simulink model "Harness_Angle"  (R2018a)
settings: Solver=VariableStepAuto  StartTime=0.0  StopTime=10.0  RelTol=1e-3
undefined symbols (not defined in the file): Automatic_Test
libraries: mciapi_libbrowser x1
settings Model: Creator=PATILMP  LastModifiedBy=PATILMP

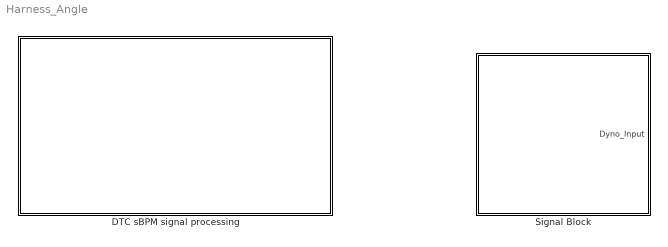
== system Harness_Angle ==
  DTC sBPM signal processing : Subsystem
  Signal Block : Subsystem

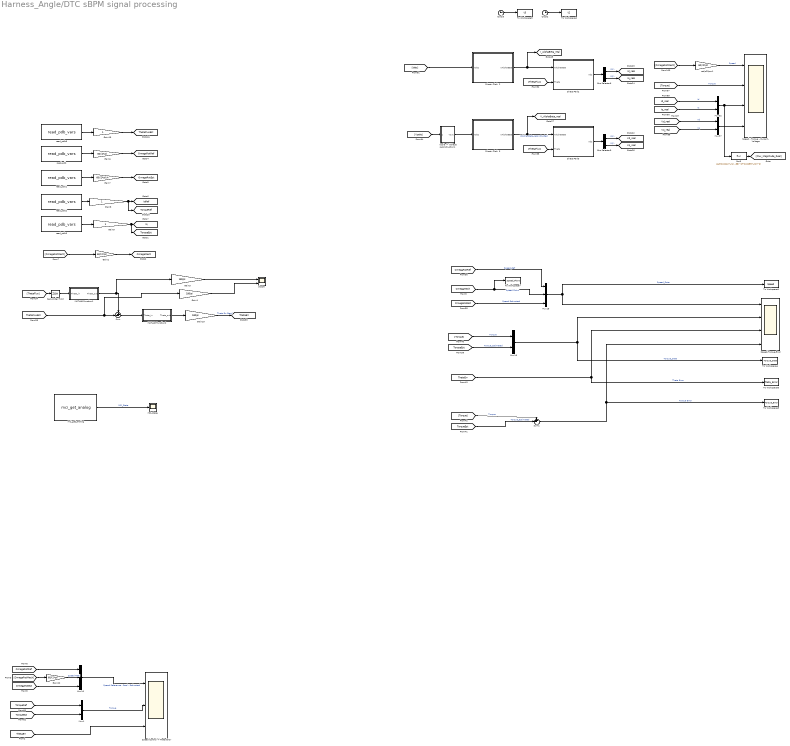
== system Harness_Angle/DTC sBPM signal processing ==
  Bus Selector6 : BusSelector  OutputSignals=D,Q
  Bus Selector9 : BusSelector  OutputSignals=D,Q
  Clock2 : Clock
  Clock3 : Clock
  Direct  Clark  2 : MATLAB Function  TreatAsAtomicUnit=on  SystemSampleTime=SystemSampleTime  mask{SystemSampleTime=-1}
      mask prompts: SystemSampleTime "Simulink:blkprm_prompts:AllBlksSampleTime"
  Direct  Clark  3 : MATLAB Function  TreatAsAtomicUnit=on  SystemSampleTime=SystemSampleTime  mask{SystemSampleTime=-1}
      mask prompts: SystemSampleTime "Simulink:blkprm_prompts:AllBlksSampleTime"
  Direct Park2 : MATLAB Function  TreatAsAtomicUnit=on  SystemSampleTime=SystemSampleTime  mask{SystemSampleTime=-1}
      mask prompts: SystemSampleTime "Simulink:blkprm_prompts:AllBlksSampleTime"
  Direct Park3 : MATLAB Function  TreatAsAtomicUnit=on  SystemSampleTime=SystemSampleTime  mask{SystemSampleTime=-1}
      mask prompts: SystemSampleTime "Simulink:blkprm_prompts:AllBlksSampleTime"
  Fcn5 : Fcn  Expr=sqrt((0.0212*u(1)+0.0688)^2+(0.0299*u(2))^2)
  Gain1 : Gain  Gain=180/pi
  Gain15 : Gain  OutDataTypeStr=double  RndMeth=Zero
  Gain19 : Gain  Gain=180/pi
  Gain2 : Gain  Gain=60/(2*pi)  RndMeth=Round
  Gain22 : Gain  Gain=60/(2*pi)  RndMeth=Round
  Gain3 : Gain  Gain=180/pi
  Gain6 : Gain  Gain=60/(2*pi)  OutDataTypeStr=double  RndMeth=Zero
  Gain7 : Gain  Gain=60/(2*pi)/4  OutDataTypeStr=double  RndMeth=Zero
  Gain8 : Gain  OutDataTypeStr=double  RndMeth=Zero
  Gain9 : Gain  OutDataTypeStr=double  RndMeth=Zero
  MATLAB Function1 : MATLAB Function  TreatAsAtomicUnit=on
  MATLAB Function2 : MATLAB Function  TreatAsAtomicUnit=on
  MCI_State : Scope
  Mux{1,16,32,37} (4 alike) : Mux  Inputs=2
  Mux10 : Mux  Inputs=3
  Mux15 : Mux  Inputs=3
  Scope : Scope  NumInputPorts=2
  Speed - Torque - Current - Voltage : Scope  NumInputPorts=4
  Speed Control + Theta Error : Scope  NumInputPorts=3
  Speed-Torque-Error : Scope  NumInputPorts=4
  Sum : Sum  Inputs=+-|
  Sum1 : Sum  Inputs=+-|
  To Workspace1 : ToWorkspace  VariableName=Speed  SaveFormat=Timeseries  SampleTime=-1
  To Workspace2 : ToWorkspace  VariableName=t2  SampleTime=-1
      settings: Save2DSignal=2-D array (concatenate along first dimension)
  To Workspace3 : ToWorkspace  VariableName=t3  SampleTime=-1
      settings: Save2DSignal=2-D array (concatenate along first dimension)
  To Workspace4 : ToWorkspace  VariableName=Torque_Data  SaveFormat=Timeseries  SampleTime=-1
  To Workspace5 : ToWorkspace  VariableName=Torque_Error  SaveFormat=Timeseries  SampleTime=-1
  To Workspace6 : ToWorkspace  VariableName=Theta_Error  SaveFormat=Timeseries  SampleTime=-1
  To Workspace7 : ToWorkspace  VariableName=Speed_Plant  SaveFormat=Timeseries  SampleTime=-1
  "Vpole -> Vphase reconstruction1" : MATLAB Function  TreatAsAtomicUnit=on
  Zero-Order Hold : ZeroOrderHold  SampleTime=0.000125
  mci_get_analog : S-Function  FunctionName=mci_get_analog  Parameters=read_data, choose_read_data  SFunctionDeploymentMode=off  EnableBusSupport=off  mask{choose_read_data=MCI_AI_INTERNAL_MCI_STATE, read_data=24}
      mask prompts: choose_read_data "Data to read"
      mask TypeOptions choose_read_data: MCI_AI_TARGET_SPEED_RPM_S16 | MCI_AI_SPEED_REFERENCE_RPM_S16 | MCI_AI_ACTUAL_SPEED_S16 | MCI_AI_SPEED_ERROR_RPM_S16 | MCI_AI_MEAN_SPEED_S16 | MCI_AI_RMS_MOTOR_CURRENT_S16 | MCI_AI_ACTIVE_POWER_S16 | MCI_AI_SHAFT_POWER_S16 | MCI_AI_MOTOR_TEMP_S16 | MCI_AI_STATOR_TEMP_S16 | MCI_AI_LOAD_TORQUE_S16 | MCI_AI_SHAFT_POSITION_DEG_S16 | MCI_AI_BUS_CURRENT_S16 | MCI_AI_BUS_VOLTAGE_S16 | MCI_AI_INVERTER_TEMP_S16 | MCI_AI_INVERTER_TEMP_RAW_DATA | MCI_AI_VOLTAGE_PHASE_A_S16 | MCI_AI_VOLTAGE_PHASE_B_S16 | MCI_AI_VOLTAGE_PHASE_C_S16 | MCI_AI_SPEED_LOOP_GAIN_TABLE_INDEX | MCI_AI_CURR_PHASE_A_S16 | MCI_AI_CURR_PHASE_B_S16 | MCI_AI_CURR_PHASE_C_S16 | MCI_AI_STATOR_RESISTANCE_S16 | MCI_AI_INTERNAL_MCI_STATE
      mask Callback read_data:
      | rd = get_param(gcb,'choose_read_data');
      | poenum = strcat('MCI_AI_TYPE.',rd);
      | i_32 = eval(['int32(' poenum ')']);
      | set_param(gcb,'read_data',int2str(i_32));
      mask Display:
      | disp = regexp(choose_read_data, 'MCI_AI_', 'split');
      | port_label('output', 1, disp{2});
  rad/s2Rpm1 : Gain  Gain=60/(2*pi)
  read_pdb : S-Function  FunctionName=read_pdb_vars  Parameters=vstring  SFunctionDeploymentMode=off  EnableBusSupport=off  mask{vstring=Mcl_IO.Speed_Rot_Ref}
      mask prompts: vstring "Variable to read"
      mask Display:
      | disp = vstring;
      | port_label('output', 1, disp);
  read_pdb1 : S-Function  FunctionName=read_pdb_vars  Parameters=vstring  SFunctionDeploymentMode=off  EnableBusSupport=off  mask{vstring=Mcl_Quantities.Speed_Rot}
      mask prompts: vstring "Variable to read"
      mask Display:
      | disp = vstring;
      | port_label('output', 1, disp);
  read_pdb2 : S-Function  FunctionName=read_pdb_vars  Parameters=vstring  SFunctionDeploymentMode=off  EnableBusSupport=off  mask{vstring=Mcl_Quantities.Torque_Ref}
      mask prompts: vstring "Variable to read"
      mask Display:
      | disp = vstring;
      | port_label('output', 1, disp);
  read_pdb3 : S-Function  FunctionName=read_pdb_vars  Parameters=vstring  SFunctionDeploymentMode=off  EnableBusSupport=off  mask{vstring=Mcl_Quantities.Torque}
      mask prompts: vstring "Variable to read"
      mask Display:
      | disp = vstring;
      | port_label('output', 1, disp);
  read_pdb8 : S-Function  FunctionName=read_pdb_vars  Parameters=vstring  SFunctionDeploymentMode=off  EnableBusSupport=off  mask{vstring=Mcl_Quantities.Rotor_Position}
      mask prompts: vstring "Variable to read"
      mask Display:
      | disp = vstring;
      | port_label('output', 1, disp);
  tag scope: I_AlphaBeta_real=global, Id_real=global, Iq=global, IqRef=global, Iq_real=global, OmegaMech=global, OmegaRotEst=global, OmegaRotRef=global, ThetaErr=global, ThetaFluxEst=global, TorqueEst=global, TorqueRef=global, V_AlphaBeta_real=global, Vd_real=global, Vq_real=global
  wires:
  [ThetaFlux] -> Zero-Order Hold/1
  MATLAB Function1/1(Theta_out) -> Gain3/1, Sum/1
  Sum/1 -> MATLAB Function2/1(Theta_in)
  Gain19/1 -> [ThetaErr]  "Theta Err [deg]"
  MATLAB Function2/1(Theta_out) -> Gain19/1
  Zero-Order Hold/1 -> MATLAB Function1/1(Theta_in)
  [ThetaFluxEst] -> Gain1/1, Sum/2
  Bus Selector6/1 -> [Id_real]  "<D>"
  [Vpole] -> "Vpole -> Vphase reconstruction1"/1(Vpole)
  [Vq_real] -> Mux37/2  "Vq"
  Bus Selector6/2 -> [Iq_real]  "<Q>"
  "Vpole -> Vphase reconstruction1"/1(Vout) -> Direct  Clark  3/1(Xabc)
  [ThetaFlux] -> Direct Park3/2(Theta)
  Mux32/1 -> Fcn5/1, Speed - Torque - Current - Voltage/3
  Direct Park2/1(Xdq) -> Bus Selector6/1
  Clock2/1 -> To Workspace2/1
  [Iq_real] -> Mux32/2  "Iq"
  rad/s2Rpm1/1 -> Speed - Torque - Current - Voltage/1  "Speed"
  Mux37/1 -> Speed - Torque - Current - Voltage/4
  Clock3/1 -> To Workspace3/1
  [Iabc] -> Direct  Clark  2/1(Xabc)
  Bus Selector9/1 -> [Vd_real]  "<D>"
  [ThetaFlux] -> Direct Park2/2(Theta)
  [Torque] -> Speed - Torque - Current - Voltage/2  "Torque"
  [Id_real] -> Mux32/1  "Id"
  [Vd_real] -> Mux37/1  "Vd"
  Bus Selector9/2 -> [Vq_real]  "<Q>"
  Direct  Clark  3/1(XAlphaBeta) -> Direct Park3/1(XAlphaBeta), [V_AlphaBeta_real]  "Valpha_Beta_reconstructed"
  Direct Park3/1(Xdq) -> Bus Selector9/1
  Direct  Clark  2/1(XAlphaBeta) -> [I_AlphaBeta_real], Direct Park2/1(XAlphaBeta)
  [OmegaRotMech] -> rad/s2Rpm1/1
  Gain8/1 -> [TorqueRef], [IqRef]
  Gain9/1 -> [TorqueEst], [Iq]
  read_pdb/1 -> Gain6/1
  read_pdb8/1 -> Gain15/1
  Gain15/1 -> [ThetaFluxEst]
  read_pdb3/1 -> Gain9/1
  read_pdb2/1 -> Gain8/1
  Gain6/1 -> [OmegaRotRef]
  read_pdb1/1 -> Gain7/1
  Gain7/1 -> [OmegaRotEst]
  [TorqueEst] -> Mux1/2
  [TorqueRef] -> Mux1/1
  Mux1/1 -> Speed Control + Theta Error/2  "Torque"
  mci_get_analog/1 -> MCI_State/1  "MCI_State"
  Fcn5/1 -> [Flux_Magnitude_Real]
  Mux15/1 -> Speed-Torque-Error/1, To Workspace1/1  "Speed_Data"
  [TorqueEst] -> Sum1/2  "Torque_estimated"
  [TorqueEst] -> Mux16/2  "Torque_estimated"
  [Torque] -> Mux16/1  "Torque"
  Sum1/1 -> Speed-Torque-Error/4, To Workspace5/1  "Torque Error"
  [OmegaRotEst] -> Mux15/3  "Speed Estimated"
  [OmegaMech] -> To Workspace7/1, Mux15/2  "Speed Plant"
  [Torque] -> Sum1/1  "Torque"
  Mux16/1 -> To Workspace4/1, Speed-Torque-Error/2  "Torque_Data"
  [ThetaErr] -> To Workspace6/1, Speed-Torque-Error/3  "Theta Error"
  [OmegaRotRef] -> Mux15/1  "Speed_Ref"
  [OmegaRotEst] -> Mux10/3
  Gain22/1 -> Mux10/2  "Speed Real"
  [OmegaRotRef] -> Mux10/1
  Mux10/1 -> Speed Control + Theta Error/1  "Speed Reference - Real - Estimated"
  [OmegaRotMech] -> Gain22/1
  [ThetaErr] -> Speed Control + Theta Error/3
  Gain2/1 -> [OmegaMech]
  [OmegaRotMech] -> Gain2/1
  Gain1/1 -> Scope/2
  Gain3/1 -> Scope/1

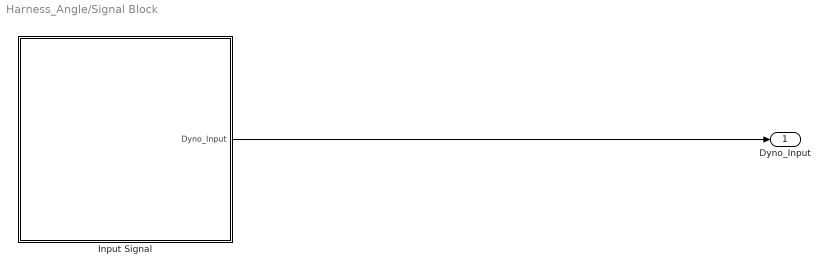
== system Harness_Angle/Signal Block ==
  Input Signal : Subsystem
  Dyno_Input : Outport
  wires:
  Input Signal/1(Dyno_Input) -> Dyno_Input/1

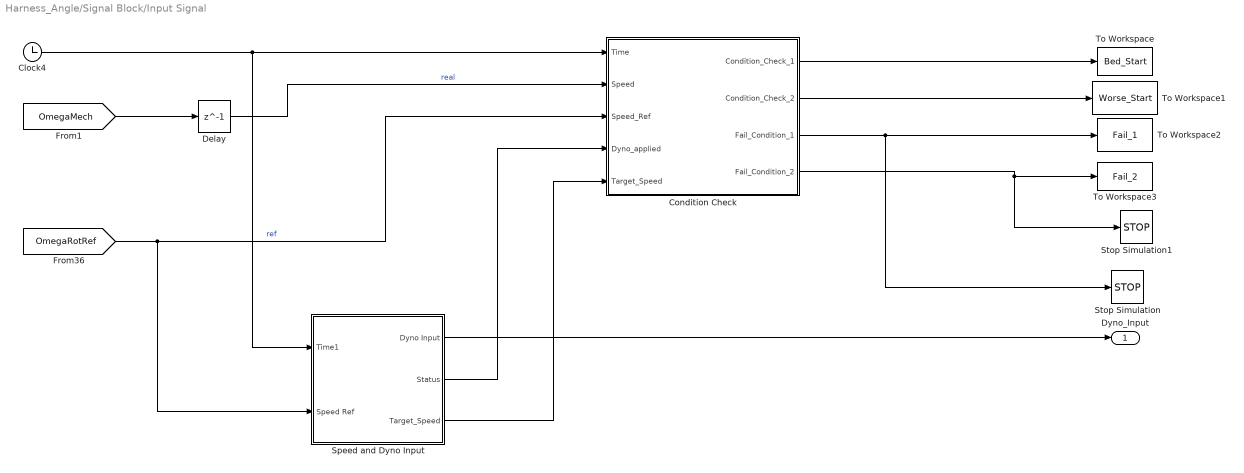
== system Harness_Angle/Signal Block/Input Signal ==
  Clock4 : Clock
  Condition Check : MATLAB Function  TreatAsAtomicUnit=on  mask(Condition Check){Speed_Tolerance=Automatic_Test.Speed_Tolerance, Para_time_check_1=Automatic_Test.Para_time_check_1, Para_time_check_2=Automatic_Test.Para_time_check_2, Para_time_check_3=Automatic_Test.Para_time_check_3, Speed_Tolerance_1=Automatic_Test.Speed_Tolerance_1}
      mask prompts: Speed_Tolerance "Speed Tolerance Value"; Speed_Tolerance_1 "Speed Tolerance Value_1"
      mask help: This block is used to check failure conditions.
  Delay : Delay  DelayLength=1
  Speed and Dyno Input : Subsystem
  Stop Simulation : Stop
  Stop Simulation1 : Stop
  To Workspace : ToWorkspace  VariableName=Bed_Start  SaveFormat=Timeseries  SampleTime=-1
  To Workspace1 : ToWorkspace  VariableName=Worse_Start  SaveFormat=Timeseries  SampleTime=-1
  To Workspace2 : ToWorkspace  VariableName=Fail_1  SaveFormat=Timeseries  SampleTime=-1
  To Workspace3 : ToWorkspace  VariableName=Fail_2  SaveFormat=Timeseries  SampleTime=-1
  Dyno_Input : Outport
  wires:
  [OmegaMech] -> Delay/1
  Delay/1 -> Condition Check/2(Speed)  "real"
  [OmegaRotRef] -> Speed and Dyno Input/2(Speed Ref), Condition Check/3(Speed_Ref)  "ref"
  Speed and Dyno Input/1(Dyno Input) -> Dyno_Input/1
  Condition Check/1(Condition_Check_1) -> To Workspace/1
  Condition Check/2(Condition_Check_2) -> To Workspace1/1
  Condition Check/3(Fail_Condition_1) -> Stop Simulation/1, To Workspace2/1
  Clock4/1 -> Condition Check/1(Time), Speed and Dyno Input/1(Time1)
  Condition Check/4(Fail_Condition_2) -> Stop Simulation1/1, To Workspace3/1
  Speed and Dyno Input/2(Status) -> Condition Check/4(Dyno_applied)
  Speed and Dyno Input/3(Target_Speed) -> Condition Check/5(Target_Speed)

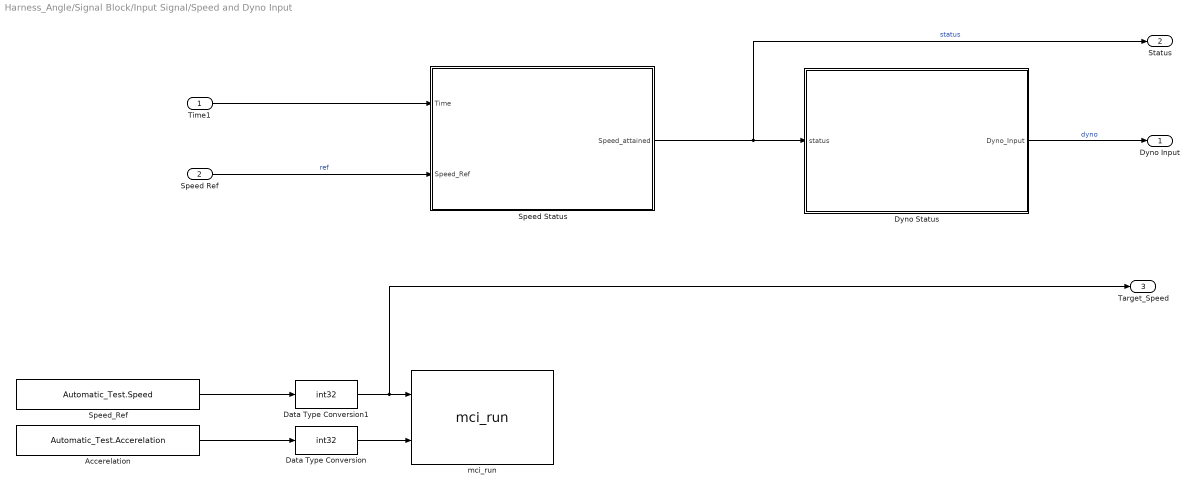
== system Harness_Angle/Signal Block/Input Signal/Speed and Dyno Input ==
  Time1 : Inport
  Speed Ref : Inport  Port=2
  Accerelation : Constant  Value=Automatic_Test.Accerelation
  Data Type Conversion : DataTypeConversion  OutDataTypeStr=int32
  Data Type Conversion1 : DataTypeConversion  OutDataTypeStr=int32
  Dyno Status : MATLAB Function  TreatAsAtomicUnit=on  mask(Speed Status){Dyno_Load=Automatic_Test.Dyno_Load}
      mask help: Once this block gets the active high signal from the speed ref status block, dyno load torque input gets activated and given as output.
  Speed Status : MATLAB Function  TreatAsAtomicUnit=on  mask(Speed Status){Status_Time_Check=Automatic_Test.Status_Time_Check}
      mask prompts: Status_Time_Check "Status Time Check"
      mask help: This Matlab function block is used to get the status of reference and estimated speed.
  Speed_Ref : Constant  Value=Automatic_Test.Speed
  mci_run : mciapi_libbrowser/mci_run  SFunctionModules=''
      settings: SourceProductName=Sim Arch
  Dyno Input : Outport
  Status : Outport  Port=2
  Target_Speed : Outport  Port=3
  wires:
  Accerelation/1 -> Data Type Conversion/1
  Data Type Conversion/1 -> mci_run/2
  Time1/1 -> Speed Status/1(Time)
  Speed Status/1(Speed_attained) -> Status/1, Dyno Status/1(status)  "status"
  Speed Ref/1 -> Speed Status/2(Speed_Ref)  "ref"
  Data Type Conversion1/1 -> Target_Speed/1, mci_run/1
  Dyno Status/1(Dyno_Input) -> Dyno Input/1  "dyno"
  Speed_Ref/1 -> Data Type Conversion1/1

== matlab function Harness_Angle/DTC sBPM signal processing/Direct  Clark  2 ==
  data: XAlphaBeta output Bus: XAlphaBetaBus; Xabc input Bus: XabcBus
function XAlphaBeta = DirectClark(Xabc)

XAlphaBeta.Alpha = Xabc.A;
XAlphaBeta.Beta =  sqrt(3)/3*(Xabc.A+2*Xabc.B);

== matlab function Harness_Angle/DTC sBPM signal processing/Direct  Clark  3 ==
  data: XAlphaBeta output Bus: XAlphaBetaBus; Xabc input Bus: XabcBus
function XAlphaBeta = DirectClark(Xabc)

XAlphaBeta.Alpha = Xabc.A;
XAlphaBeta.Beta =  sqrt(3)/3*(Xabc.A+2*Xabc.B);

== matlab function Harness_Angle/DTC sBPM signal processing/Direct Park2 ==
  data: XAlphaBeta input Bus: XAlphaBetaBus; Xdq output Bus: XdqBus; Theta input
function Xdq = DirectPark(XAlphaBeta,Theta)

Xdq.D  =  XAlphaBeta.Alpha*cos(Theta) + XAlphaBeta.Beta*sin(Theta);
Xdq.Q  = -XAlphaBeta.Alpha*sin(Theta) + XAlphaBeta.Beta*cos(Theta);

== matlab function Harness_Angle/DTC sBPM signal processing/Direct Park3 ==
  data: XAlphaBeta input Bus: XAlphaBetaBus; Xdq output Bus: XdqBus; Theta input
function Xdq = DirectPark(XAlphaBeta,Theta)

Xdq.D  =  XAlphaBeta.Alpha*cos(Theta) + XAlphaBeta.Beta*sin(Theta);
Xdq.Q  = -XAlphaBeta.Alpha*sin(Theta) + XAlphaBeta.Beta*cos(Theta);

== matlab function Harness_Angle/DTC sBPM signal processing/MATLAB Function1 ==
  data: Theta_in input; Theta_out output
function Theta_out = fcn(Theta_in)
%#codegen

if(Theta_in > pi)||(Theta_in < -pi)
    
    Resto_pi =  mod(Theta_in, pi);
    Resto_2pi =  mod(Theta_in, 2*pi);
    
    
    if(Resto_pi ~= Resto_2pi)
    Theta_out = -pi+Resto_pi;
    else
    Theta_out = Resto_pi;    
    end
 
else
    
    Theta_out = Theta_in;
    
end

== matlab function Harness_Angle/DTC sBPM signal processing/MATLAB Function2 ==
  data: Theta_in input; Theta_out output
function Theta_out = fcn(Theta_in)
%#codegen

if(Theta_in > pi)||(Theta_in < -pi)
    
    Resto_pi =  mod(Theta_in, pi);
    Resto_2pi =  mod(Theta_in, 2*pi);
    
    
    if(Resto_pi ~= Resto_2pi)
    Theta_out = -pi+Resto_pi;
    else
    Theta_out = Resto_pi;    
    end
 
else
    
    Theta_out = Theta_in;
    
end

== matlab function Harness_Angle/DTC sBPM signal processing/Vpole -> Vphase reconstruction1 ==
  data: Vpole input Bus: XabcBus size=1; Vout output Bus: XabcBus
function Vout   = Vrec2(Vpole)

Va = Vpole.A;
Vb = Vpole.B;
Vc = Vpole.C;

Vn = (Va + Vb + Vc)/3;

Vphase.A = Va - Vn;
Vphase.B = Vb - Vn;
Vphase.C = Vc - Vn;

Vline.A = Va - Vb;  % Vab
Vline.B = Vb - Vc;  % Vbc
Vline.C = Vc - Va;  % Vca

Vout = Vphase;
end

== matlab function Harness_Angle/Signal Block/Input Signal/Condition Check ==
  data: Condition_Check_1 output; Condition_Check_2 output; Fail_Condition_1 output; Time input; Speed input; Speed_Ref input; Dyno_applied input; Target_Speed input; Speed_Tolerance parameter; Para_time_check_1 parameter; Para_time_check_2 parameter; Para_time_check_3 parameter; Speed_Tolerance_1 parameter; Fail_Condition_2 output
function [Condition_Check_1,Condition_Check_2,Fail_Condition_1,Fail_Condition_2] = fcn(Time,Speed,Speed_Ref,Dyno_applied,Target_Speed,Speed_Tolerance,Para_time_check_1,Para_time_check_2,Para_time_check_3,Speed_Tolerance_1)

persistent old_value1
persistent old_value2
persistent old_value3
persistent count

if isempty(old_value1)
    old_value1=0;
end
if isempty(old_value2)
    old_value2=0;
end
if isempty(old_value3)
    old_value3=0;
end

if isempty(count)
    count=0;
end

ST=Speed_Tolerance/100;
ST1=Speed_Tolerance_1/100;
Limit=Speed_Ref*ST;
Delta_Speed=abs(Speed-Speed_Ref);

Fail_Condition_1=0;
Fail_Condition_2=0;
Condition_Check_1 = 0;
Condition_Check_2 = 0;

if Dyno_applied==1
 if (Delta_Speed > Limit)
        if((Time-old_value1)>Para_time_check_2)
             Fail_Condition_1= 1;  
        elseif((Time-old_value2)>Para_time_check_1)
            count = count+1;
            old_value2 = Time; 
         end
 else
        old_value1 = Time;
 end 
end

 if int32(Speed_Ref) >= Target_Speed
     old_value3 = Time;
     if (Speed>= Speed_Ref+ST1*Speed_Ref)
    if(old_value3> Para_time_check_3)
    Fail_Condition_2= 1;
    end
     end
if count > 1
    Condition_Check_2 = 1; 
elseif(count==1)
    Condition_Check_1 = 1; 
else
Condition_Check_1 = 0;
Condition_Check_2 = 0;
    
end

end

== matlab function Harness_Angle/Signal Block/Input Signal/Speed and Dyno Input/Dyno Status ==
  data: Dyno_Input output; status input; Dyno_Load parameter
function Dyno_Input= fcn(status,Dyno_Load)
if status==1
    Dyno_Input=Dyno_Load;
else
   Dyno_Input=0 ;      
end

== matlab function Harness_Angle/Signal Block/Input Signal/Speed and Dyno Input/Speed Status ==
  data: Speed_attained output; Time input; Speed_Ref input; Status_Time_Check parameter
function Speed_attained = fcn(Time,Speed_Ref,Status_Time_Check)
persistent t_old
persistent flag


if isempty(t_old)
    t_old =0;
end

if isempty(flag)
    flag = 0;
end

if abs(Speed_Ref)~=0
   flag = 1;
end

if flag == 0
    t_old = Time;
end

if (Time-t_old)>Status_Time_Check
    Speed_attained = 1;
else
    Speed_attained = 0;
end
